simulink model "open_loop"  (R2015a)
settings: Solver=ode4  StartTime=0.0  StopTime=20  FixedStep=0.01  MaxStep=0.01  RelTol=1e-3
libraries: mblibv1 x10
settings Model: Creator=peixeboi  LastModifiedBy=peixeboi
settings SolverCC: ZeroCrossControl=DisableAll

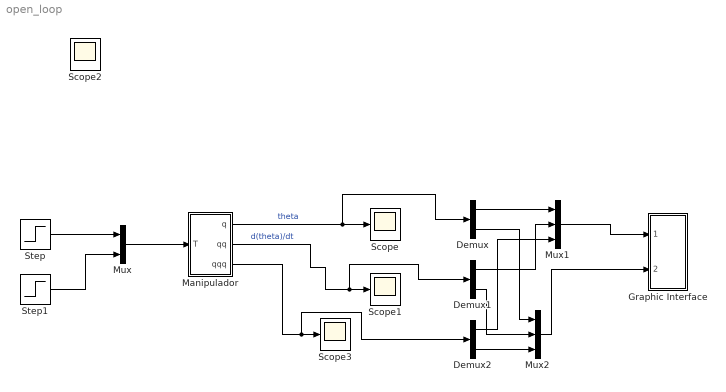
== system open_loop ==
  Demux : Demux  Outputs=2
  Demux1 : Demux  Outputs=2
  Demux2 : Demux  Outputs=2
  Graphic Interface : Subsystem
  Manipulador : Subsystem
  Mux : Mux  Inputs=2
  Mux1 : Mux  Inputs=3
  Mux2 : Mux  Inputs=3
  Scope{,1..3} (4 alike) : Scope
      Scope settings: ShowLegends=on
      Scope1 settings: ShowLegends=on
      Scope3 settings: ShowLegends=on  SaveName=ScopeData3
      Scope2 settings: SaveName=ScopeData2
  Step : Step  Time=0  After=0  SampleTime=0
  Step1 : Step  Time=0  After=0  SampleTime=0
  wires:
  Mux/1 -> Manipulador/1(T)
  Manipulador/2(qq) -> Demux1/1, Scope1/1  "d(theta)/dt"
  Manipulador/1(q) -> Demux/1, Scope/1  "theta"
  Step/1 -> Mux/1
  Step1/1 -> Mux/2
  Mux1/1 -> Graphic Interface/1(theta1)
  Demux/1 -> Mux1/1
  Mux2/1 -> Graphic Interface/2(theta2)
  Demux/2 -> Mux2/1
  Demux1/1 -> Mux1/2
  Demux2/1 -> Mux1/3
  Demux1/2 -> Mux2/2
  Demux2/2 -> Mux2/3
  Manipulador/3(qqq) -> Demux2/1, Scope3/1

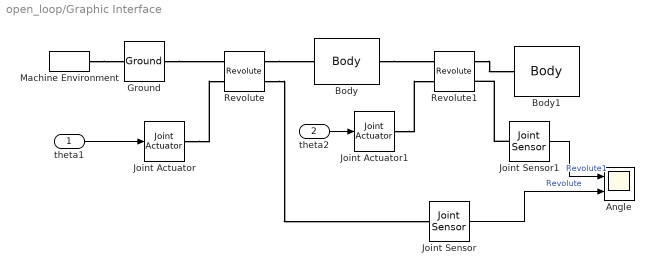
== system open_loop/Graphic Interface ==
  theta1 : Inport
  theta2 : Inport  Port=2
  Angle : Scope  NumInputPorts=2
      settings: TimeRange=10  YMin=-120~-1  YMax=0~1
  Body : mblibv1/Bodies/Body  LConnTagsString=CS1  RConnTagsString=CS2  UpdateFromCAD=off  DialogClass=MechanicalBodyBlock  Mass=2.2  MassUnits=kg  InertiaUnits=kg*m^2  Inertia=[0.565529 0 0; 0 0.00085 0; 0 0 0.565529]  Shape=Cylinder  ShapeDims=[1 1]  ShapeUnits=m  ShapeUse=false  Density=1  DensityUnits=kg/m^3  DensityUse=false  GraphicsMode=MACHINE_DEFAULT  BodyColorSelMode=MACHINE_DEFAULT  BodyColor=[1 0 0]  AttachedToCS=CG  CG=Left$CG$[0.3 0 0]$WORLD$WORLD$m$[0 0 pi/4]$Euler X-Y-Z$rad$WORLD$false$none  WorkingFrames=Left$CS1$[0 0 0]$WORLD$WORLD$m$[0 0 0]$Euler X-Y-Z$deg$WORLD$true$none#Right$CS2$[0.6 0 0]$WORLD$WORLD$m$[0 0 0]$Euler X-Y-Z$deg$WORLD$true$none  CGPos=[0.3 0 0]  CGRot=[0 0 pi/4]  CS0Pos=[]  CS0Rot=[]  CS1Pos=[0 0 0]  CS1Rot=[0 0 0]  CS2Pos=[0.6 0 0]  CS2Rot=[0 0 0]  CS3Pos=[]  CS3Rot=[]  CS4Pos=[]  CS4Rot=[]  CS5Pos=[]  CS5Rot=[]  CS6Pos=[]  CS6Rot=[]  CS7Pos=[]  CS7Rot=[]  CS8Pos=[]  CS8Rot=[]  CS9Pos=[]  CS9Rot=[]  CS10Pos=[]  CS10Rot=[]  CS11Pos=[]  CS11Rot=[]  CS12Pos=[]  CS12Rot=[]  CS13Pos=[]  CS13Rot=[]  CS14Pos=[]  CS14Rot=[]  CS15Pos=[]  CS15Rot=[]  CS16Pos=[]  CS16Rot=[]  CS17Pos=[]  CS17Rot=[]  CS18Pos=[]  CS18Rot=[]  CS19Pos=[]  CS19Rot=[]  CS20Pos=[]  CS20Rot=[]
  Body1 : mblibv1/Bodies/Body  LConnTagsString=CS1  UpdateFromCAD=off  DialogClass=MechanicalBodyBlock  Mass=2.2  MassUnits=kg  InertiaUnits=kg*m^2  Inertia=[0.565529 0 0; 0 0.00085 0; 0 0 0.565529]  Shape=Cylinder  ShapeDims=[1 1]  ShapeUnits=m  ShapeUse=false  Density=1  DensityUnits=kg/m^3  DensityUse=false  GraphicsMode=MACHINE_DEFAULT  BodyColorSelMode=MACHINE_DEFAULT  BodyColor=[1 0 0]  AttachedToCS=CG  CG=Left$CG$[0.9 0 0]$WORLD$WORLD$m$[0 0 pi/4]$Euler X-Y-Z$rad$WORLD$false$none  WorkingFrames=Left$CS1$[0.6 0 0]$WORLD$WORLD$m$[0 0 0]$Euler X-Y-Z$deg$WORLD$true$none#Right$CS2$[1.2 0 0]$WORLD$WORLD$m$[0 0 0]$Euler X-Y-Z$deg$WORLD$false$none  CGPos=[0.9 0 0]  CGRot=[0 0 pi/4]  CS0Pos=[]  CS0Rot=[]  CS1Pos=[0.6 0 0]  CS1Rot=[0 0 0]  CS2Pos=[1.2 0 0]  CS2Rot=[0 0 0]  CS3Pos=[]  CS3Rot=[]  CS4Pos=[]  CS4Rot=[]  CS5Pos=[]  CS5Rot=[]  CS6Pos=[]  CS6Rot=[]  CS7Pos=[]  CS7Rot=[]  CS8Pos=[]  CS8Rot=[]  CS9Pos=[]  CS9Rot=[]  CS10Pos=[]  CS10Rot=[]  CS11Pos=[]  CS11Rot=[]  CS12Pos=[]  CS12Rot=[]  CS13Pos=[]  CS13Rot=[]  CS14Pos=[]  CS14Rot=[]  CS15Pos=[]  CS15Rot=[]  CS16Pos=[]  CS16Rot=[]  CS17Pos=[]  CS17Rot=[]  CS18Pos=[]  CS18Rot=[]  CS19Pos=[]  CS19Rot=[]  CS20Pos=[]  CS20Rot=[]
  Ground : mblibv1/Bodies/Ground  UpdateFromCAD=off  LeftPortType=env  RightPortType=workingframe  PhysicalDomain=Mechanical  DialogClass=GroundBlock  CoordPosition=[0 0 0]  CoordPositionUnits=m  StateVectorMgrId=0  MachineId=[1 0]  ShowEnvPort=on  ParameterChecksum=[2665323517, 9994337, 2049993874, 3484898119]  TopologyChecksum=[3214554247, 653845476, 1212418715, 3884345933]
  Joint Actuator : mblibv1/Sensors &  Actuators/Joint Actuator  UpdateFromCAD=off  PhysicalDomain=Mechanical  PortType=blob  ActuationStyle=Motion  AngleUnits=rad  ArcVelocityUnits=rad/s  ArcAccelerationUnits=rad/s^2  CoordPositionUnits=m  VelocityUnits=m/s  AccelerationUnits=m/s^2  ForceUnits=N  TorqueUnits=N*m  ActiveIO=on  Width=3  DialogClass=MechanicalActuatorBlock  Primitive=R1  ReferenceFrame=Absolute (INERTIAL)
  Joint Actuator1 : mblibv1/Sensors &  Actuators/Joint Actuator  UpdateFromCAD=off  PhysicalDomain=Mechanical  PortType=blob  ActuationStyle=Motion  AngleUnits=rad  ArcVelocityUnits=rad/s  ArcAccelerationUnits=rad/s^2  CoordPositionUnits=m  VelocityUnits=m/s  AccelerationUnits=m/s^2  ForceUnits=N  TorqueUnits=N*m  ActiveIO=on  Width=3  DialogClass=MechanicalActuatorBlock  Primitive=R1  ReferenceFrame=Absolute (INERTIAL)
  Joint Sensor : mblibv1/Sensors &  Actuators/Joint Sensor  UpdateFromCAD=off  PhysicalDomain=Mechanical  PortType=blob  Muxed=on  Pose=on  Angle=on  AngleUnits=rad  ArcVelocity=off  ArcVelocityUnits=deg/s  ArcAcceleration=off  ArcAccelerationUnits=deg/s^2  CoordPosition=on  CoordPositionUnits=m  Velocity=off  VelocityUnits=m/s  Acceleration=off  AccelerationUnits=m/s^2  Quaternion=on  QuaternionDT=off  QuaternionDDT=off  QuaternionUnits=off  OutputVector=[1]  ActiveIO=on  Width=1  DialogClass=MechanicalSensorBlock  Primitive=R1  Force=off  ForceUnits=N  Torque=off  TorqueUnits=N*m  ReferenceFrame=Absolute (INERTIAL)  ReactionSensedSide=Base  ReactionReferenceFrame=Absolute (World)  ReactionForce=off  ReactionForceUnits=N  ReactionMoment=off  ReactionMomentUnits=N*m
  Joint Sensor1 : mblibv1/Sensors &  Actuators/Joint Sensor  UpdateFromCAD=off  PhysicalDomain=Mechanical  PortType=blob  Muxed=on  Pose=on  Angle=on  AngleUnits=rad  ArcVelocity=off  ArcVelocityUnits=deg/s  ArcAcceleration=off  ArcAccelerationUnits=deg/s^2  CoordPosition=on  CoordPositionUnits=m  Velocity=off  VelocityUnits=m/s  Acceleration=off  AccelerationUnits=m/s^2  Quaternion=on  QuaternionDT=off  QuaternionDDT=off  QuaternionUnits=off  OutputVector=[1]  ActiveIO=on  Width=1  DialogClass=MechanicalSensorBlock  Primitive=R1  Force=off  ForceUnits=N  Torque=off  TorqueUnits=N*m  ReferenceFrame=Absolute (INERTIAL)  ReactionSensedSide=Base  ReactionReferenceFrame=Absolute (World)  ReactionForce=off  ReactionForceUnits=N  ReactionMoment=off  ReactionMomentUnits=N*m
  Machine Environment : mblibv1/Bodies/Machine Environment  Tag=Factory ground  PortType=env  PhysicalDomain=Mechanical  DialogTemplateClass=MECH.MachineEnvironment  SyncWhenCopied=off  Gravity=[0 -9.81 0]  GravityUnits=m/s^2  GravityAsSignal=off  Dimensionality=3D Only  AnalysisType=Forward dynamics  LinearAssemblyTolerance=1e-3  LinearAssemblyToleranceUnits=m  AngularAssemblyTolerance=1e-3  AngularAssemblyToleranceUnits=rad  ConstraintSolverType=Stabilizing  ConstraintRelTolerance=1e-4  ConstraintAbsTolerance=1e-4  UseRobustSingularityHandling=off  RedundancyAnalysisToleranceType=Automatically select tolerance  RedundancyAnalysisTolerance=1e-14  StatePerturbationType=Adaptive  PerturbationSize=1e-3  VisualizeMachine=on  BodyVisualizationType=Use model default body geometries  BodyColorSelMode=Use model default  DefaultBodyColor=[1 0 0]
  Revolute : mblibv1/Joints/Revolute  LConnTagsString=__newl0|SA1  RConnTagsString=__newr0|SA1  UpdateFromCAD=off  NumSAPorts=2  CutJoint=off  MarkAsCut=off  Primitives=revolute  PrimitiveProps=R1$World$[0 0 1]$revolute  DialogClass=JointBlock  R1Axis=[0 0 1]
  Revolute1 : mblibv1/Joints/Revolute  LConnTagsString=__newl0|SA1  RConnTagsString=__newr0|SA1  UpdateFromCAD=off  NumSAPorts=2  CutJoint=off  MarkAsCut=off  Primitives=revolute  PrimitiveProps=R1$WORLD$[0 0 1]$revolute  DialogClass=JointBlock  R1Axis=[0 0 1]
  wires:
  theta1/1 -> Joint Actuator/1
  theta2/1 -> Joint Actuator1/1
  Joint Sensor/1 -> Angle/2  "Revolute"
  Joint Sensor1/1 -> Angle/1  "Revolute1"
  connections:
  Joint Sensor1/LConn1 -- Revolute1/RConn2
  Revolute/RConn2 -- Joint Sensor/LConn1
  Joint Actuator1/RConn1 -- Revolute1/LConn2
  Joint Actuator/RConn1 -- Revolute/LConn2
  Ground/RConn1 -- Revolute/LConn1
  Machine Environment/RConn1 -- Ground/LConn1
  Revolute1/RConn1 -- Body1/LConn1
  Body/RConn1 -- Revolute1/LConn1
  Revolute/RConn1 -- Body/LConn1

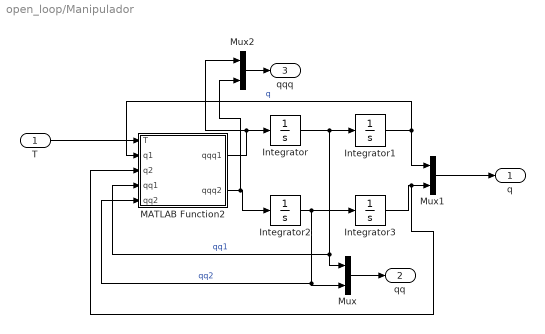
== system open_loop/Manipulador ==
  T : Inport
  Integrator : Integrator
  Integrator1 : Integrator
  Integrator2 : Integrator
  Integrator3 : Integrator  InitialCondition=pi/3
  MATLAB Function2 : MATLAB Function  TreatAsAtomicUnit=on
  Mux : Mux  Inputs=2
  Mux1 : Mux  Inputs=2
  Mux2 : Mux  Inputs=2
  q : Outport  PortDimensions=2
  qq : Outport  Port=2
  qqq : Outport  Port=3
  wires:
  Integrator/1 -> MATLAB Function2/4(qq1), Mux/1, Integrator1/1  "qq1"
  T/1 -> MATLAB Function2/1(T)
  MATLAB Function2/1(qqq1) -> Integrator/1, Mux2/1
  MATLAB Function2/2(qqq2) -> Mux2/2, Integrator2/1
  Integrator2/1 -> MATLAB Function2/5(qq2), Mux/2, Integrator3/1  "qq2"
  Mux/1 -> qq/1
  Integrator1/1 -> Mux1/1, MATLAB Function2/2(q1)  "q"
  Integrator3/1 -> MATLAB Function2/3(q2), Mux1/2
  Mux1/1 -> q/1
  Mux2/1 -> qqq/1

== matlab function open_loop/Manipulador/MATLAB Function2 ==
  data: T input; q1 input; q2 input; qqq1 output; qq1 input; qq2 input; qqq2 output
function [qqq1, qqq2] = Manip(T, q1, q2, qq1, qq2)
m1 = 2.2;
m2 = 2.2;
L1 = 0.6;
L2 = 0.6;
g=9.81;
l1 = 0.3;
l2 = 0.3;
I1 = 0.066;
I2 = 0.066;
mp=3;

H = zeros(2,1);
H(1) = -L1*(m2*l2+mp*L2)*sin(q2)*(2*qq1*qq2+qq2^2)+(m1*l1+(m2+mp)*L1)*g*cos(q1)+(m2*l2+mp*L1)*g*cos(q1+q2);
H(2) = L1*(m2*l2+mp*L2)*sin(q2)*qq1^2+(m2*l2+mp*L1)*g*cos(q1+q2);

M = zeros(2,2);
M(1,1) = I1+I2+m1*l1^2+(m2+mp)*L1^2+m2*(l2^2+L2^2)+2*L1*(m2*l2+mp*L2)*cos(q2);
M(1,2) = I2+m2*l2^2+mp*L2^2+L1*(m2*l2+mp*L2)*cos(q2);
M(2,1) = M(1,2);
M(2,2) = I2+m2*l2^2+mp*L2^2;

B = [5*qq1;
    5*qq2];

b = T - H - B; 
qqq = M\b;
qqq1 = qqq(1);
qqq2 = qqq(2);
end
